simulink model "model2020a"  (R2020b)
settings: Solver=VariableStepAuto  StartTime=0.0  StopTime=200  RelTol=1e-3
values from neighbouring files (symbols this model uses):
  A = 2.42    [constantes.m]    (also in tentandoAgain.m; testes.m)
  An = [40 25 16 12 10]    [constantes.m]    (also in tentandoAgain.m = 40; testes.m = 16)
  beta = 0.4    [constantes.m]    (also in tentandoAgain.m; testes.m)
  Cd = 0.32    [constantes.m]    (also in tentandoAgain.m; testes.m)
  Cr = 0.01    [constantes.m]    (also in tentandoAgain.m; testes.m)
  g = 9.8    [constantes.m]    (also in tentandoAgain.m; testes.m)
  M = 989    [constantes.m]    (also in tentandoAgain.m; testes.m)
  p = 1.3    [constantes.m]    (also in tentandoAgain.m; testes.m)
  Tmax = 190    [constantes.m]    (also in tentandoAgain.m; testes.m)
  Wmax = 420    [constantes.m]    (also in tentandoAgain.m; testes.m)
undefined symbols (not defined in the file or in its folder): magnitude
libraries: simulink x2
settings Model: Creator=marcelo  LastModifiedBy=joao

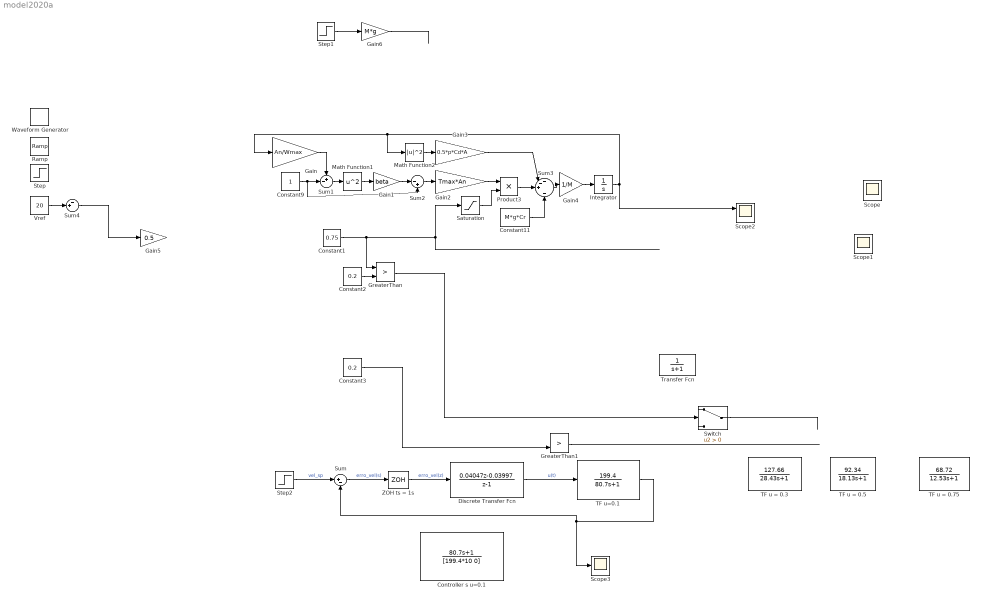
== system model2020a ==
  Constant1 : Constant  Value=0.75
  Constant11 : Constant  Value=M*g*Cr
  Constant2 : Constant  Value=0.2
  Constant3 : Constant  Value=0.2
  Constant9 : Constant
  Controller s u=0.1 : TransferFcn  Numerator=[80.7 1]  Denominator=[199.4*10 0]
  Discrete Transfer Fcn : DiscreteTransferFcn  Numerator=[0.04047 -0.03997]  Denominator=[1 -1]
  Gain : Gain  Gain=An/Wmax
  Gain1 : Gain  Gain=beta
  Gain2 : Gain  Gain=Tmax*An
  Gain3 : Gain  Gain=0.5*p*Cd*A
  Gain4 : Gain  Gain=1/M
  Gain5 : Gain  Gain=0.5
  Gain6 : Gain  Gain=M*g
  GreaterThan : RelationalOperator  Operator=>  OutDataTypeStr=boolean  RndMeth=Simplest
  GreaterThan1 : RelationalOperator  Operator=>  OutDataTypeStr=boolean  RndMeth=Simplest
  Integrator : Integrator
  Math Function1 : Math  Operator=square  SaturateOnIntegerOverflow=on
  Math Function2 : Math  Operator=magnitude^2  SaturateOnIntegerOverflow=on
  Product3 : Product
  Ramp : simulink/Sources/Ramp  slope=1  start=0  InitialOutput=0
  Saturation : Saturate  UpperLimit=1  LowerLimit=0
  Scope : Scope  NumInputPorts=3
  Scope1 : Scope  NumInputPorts=3
  Scope2 : Scope  NumInputPorts=2
  Scope3 : Scope
  Step : Step  Time=10  Before=30  After=60  SampleTime=0
  Step1 : Step  Time=5  After=-0.2  SampleTime=0
  Step2 : Step  After=55  SampleTime=0
  Sum : Sum  Inputs=|+-
  Sum1 : Sum  Inputs=+-|
  Sum2 : Sum  Inputs=|-+
  Sum3 : Sum  Inputs=--+|-
  Sum4 : Sum  Inputs=-+|
  Switch : Switch  Criteria=u2 > Threshold
  TF u = 0.3 : TransferFcn  Numerator=[127.66]  Denominator=[28.43 1]
  TF u = 0.5 : TransferFcn  Numerator=[92.34]  Denominator=[18.13 1]
  TF u = 0.75 : TransferFcn  Numerator=[68.72]  Denominator=[12.53 1]
  TF u=0.1 : TransferFcn  Numerator=[199.4]  Denominator=[80.7 1]
  Transfer Fcn : TransferFcn  Denominator=[1 1]
  Vref : Constant  Value=20
  Waveform Generator : simulink/Sources/Waveform Generator  OutMin=[]  OutMax=[]  OutDataTypeStr=double  SelectedSignal=1  Signals=sin(10, 0.5, 0)+10  BlockNames=MultiportSwitch_961ec6ff363e465  SampleTime=0.1
  ZOH ts = 1s : ZeroOrderHold
  wires:
  Integrator/1 -> Scope2/1, Math Function2/1, Gain/1
  Gain4/1 -> Integrator/1
  Constant9/1 -> Sum2/2, Sum1/2
  Gain/1 -> Sum1/1
  Sum1/1 -> Math Function1/1
  Math Function1/1 -> Gain1/1
  Gain1/1 -> Sum2/1
  Sum2/1 -> Gain2/1
  Gain2/1 -> Product3/1
  Constant1/1 -> GreaterThan/1, Saturation/1
  Math Function2/1 -> Gain3/1
  Gain3/1 -> Sum3/2
  Product3/1 -> Sum3/3
  Constant11/1 -> Sum3/4
  Sum3/1 -> Gain4/1
  Vref/1 -> Sum4/2
  Sum4/1 -> Gain5/1
  Step1/1 -> Gain6/1
  Gain6/1 -> ?
  Saturation/1 -> Product3/2
  Constant2/1 -> GreaterThan/2
  GreaterThan/1 -> Switch/2
  Switch/1 -> ?
  ? -> Switch/3
  ? -> Switch/1
  Constant3/1 -> GreaterThan1/2
  ? -> GreaterThan1/1
  GreaterThan1/1 -> ?
  ? -> Scope2/2
  Step2/1 -> Sum/1  "vel_sp"
  Sum/1 -> ZOH ts = 1s/1  "erro_vel(s)"
  TF u=0.1/1 -> Sum/2, Scope3/1
  ZOH ts = 1s/1 -> Discrete Transfer Fcn/1  "erro_vel(z)"
  Discrete Transfer Fcn/1 -> TF u=0.1/1  "u(t)"
